simulink model "environment"  (R2025a)
settings: Solver=VariableStepAuto  StartTime=0.0  StopTime=10.0  RelTol=1e-3
undefined symbols (not defined in the file or in its folder): IAU, Orbit, WMM2025
libraries: aerolibtransform2 x1, aerolibgravity2 x1
settings Model: Creator=arroy  LastModifiedBy=arroy

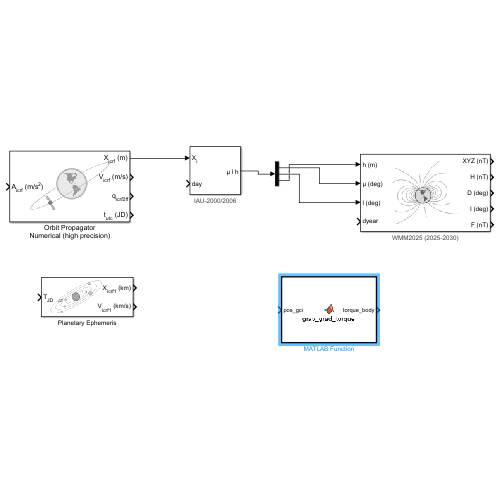
[thumbnail: Simulink's stored preview of the top-level diagram]
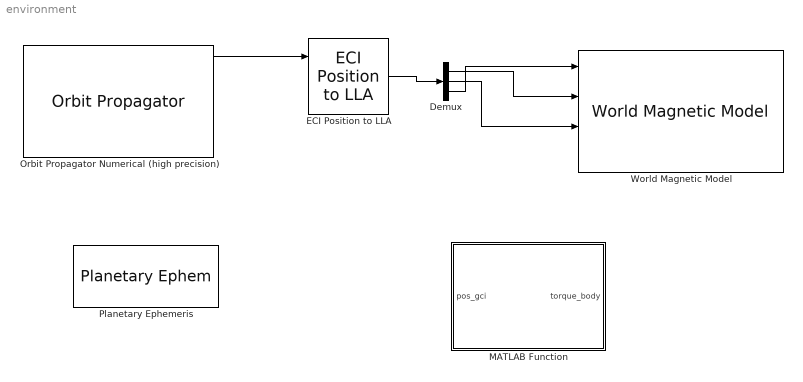
== system environment ==
  Demux : Demux  Outputs=3
  ECI Position to LLA : aerolibtransform2/ECI Position to LLA  red=IAU-2000/2006  year=2013  month=January  day=1  hour=0  min=0  sec=0  deltaT=Day  errorflag=Error  extraparamflag=off  eunits=Metric (MKS)  earthmodel=WGS84  flat=1/298.257223563  eqradius=6378137
      settings: AttributesFormatString=%<red>
  MATLAB Function : MATLAB Function  TreatAsAtomicUnit=on
  Orbit Propagator Numerical (high precision) : OrbitPropagator  propagator=Numerical (high precision)  accelIn=on  semiMajorAxis=Orbit.radius  eccentricity=Orbit.eccentricity;  inclination=Orbit.inclination  inertialPosition=[3649700.0 3308200.0 -4676600.0]  inertialVelocity=[-2750.8 6666.4 2573.4]  fixedPosition=[-4142689.0 -2676864.7 -4669861.6]  fixedVelocity=[1452.7 -6720.7 2568.1]  customR=3396200  customMu=4.305e13  customJ2=1.0826269e-03  customOmega=4.06125949e-3  outputTransform=on  useDrag=on
  Planetary Ephemeris : PlanetaryEphem
  World Magnetic Model : aerolibgravity2/World Magnetic Model  model=WMM2025 (2025-2030)  customFile='WMM2025.COF'  units=Metric (MKS)  time_in=on  month=January  day=1  year=2025  action=Error  h_out=on  dec_out=on  inc_out=on  ti_out=on
  wires:
  ECI Position to LLA/1 -> Demux/1
  Orbit Propagator Numerical (high precision)/1 -> ECI Position to LLA/1
  Demux/1 -> World Magnetic Model/2
  Demux/2 -> World Magnetic Model/3
  Demux/3 -> World Magnetic Model/1

== matlab function environment/MATLAB Function ==
  data: pos_gci input; torque_body output
function torque_body  = grav_grad_torque(pos_gci)
    % mass of earth, grav constant

    radius = norm(pos_gci);
    nadir_vec = -normalize(pos_gci);
    torque_body = cross(3*Orbit.mu/radius^3*nadir_vec, ...
        Sat.J*nadir_vec);
